simulink model "MainModel1"  (R2020a)
settings: Solver=FixedStepAuto  StartTime=0.0  StopTime=10  FixedStep=1e-3  RelTol=1e-3  EnableMultiTasking=on
undefined symbols (not defined in the file): A0, A3, D0, D1, D10, D11, D12, D13, D2, D3, D4, D5, D6, D7, D8, D9, PTA0, PTA1, PTA2, PTB11, PTB2, PTB23, PTB9, PTC16, PTC17, PTC2, PTC3, PTC4, PTD0, PTD1, PTD2, PTD3
libraries: frdmk64flib x17
settings Model: SimulationMode=external  ExtModeTrigDuration=5  Creator=prana  LastModifiedBy=prana
settings OptimizationCC: EnhancedBackFolding=on  PassReuseOutputArgsAs=Individual arguments  ZeroExternalMemoryAtStartup=off  ZeroInternalMemoryAtStartup=off  MaxStackSize=64  OptimizeBlockOrder=speed  DifferentSizesBufferReuse=on  OptimizationCustomize=off  EfficientTunableParamExpr=on
settings DebuggingCC: ParameterTunabilityLossMsg=error
settings HardwareCC: ProdBitPerPointer=32  ProdBitPerSizeT=32  ProdBitPerPtrDiffT=32  ProdLargestAtomicInteger=Long  ProdLargestAtomicFloat=Double  ProdWordSize=32  ProdHWDeviceType=ARM Compatible->ARM Cortex
settings SFSimCC: MATLABDynamicMemAlloc=off
settings RTWCC: SystemTargetFile=ert.tlc  HardwareBoard=NXP FRDM-K64F  TemplateMakefile=ert_default_tmf  Toolchain=GNU Tools for ARM Embedded Processors
settings CodeAppCC: ForceParamTrailComments=on  IgnoreCustomStorageClasses=off  OperatorAnnotations=on  SimulinkDataObjDesc=on  SFDataObjDesc=on  InsertBlockDesc=on

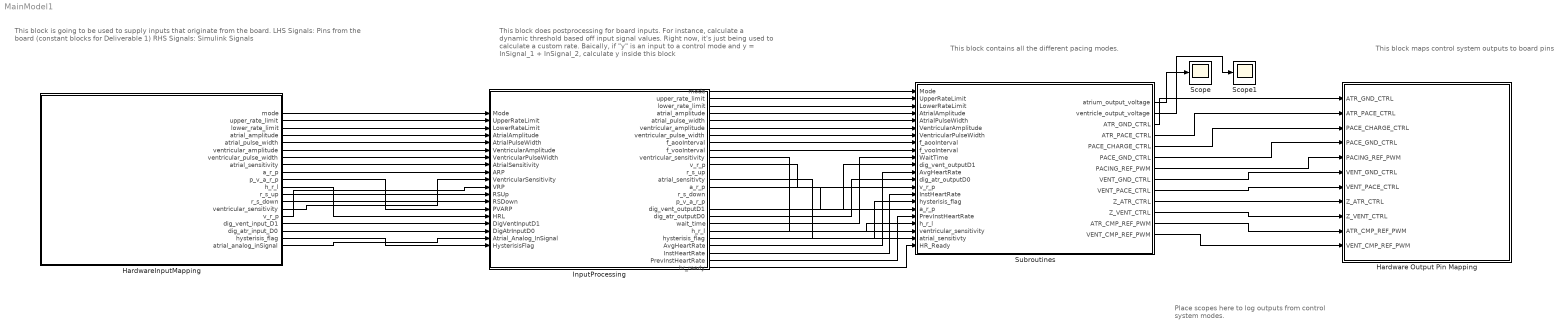
== system MainModel1 ==
  note: This block does postprocessing for board inputs.
      | For instance, calculate a dynamic threshold based off input signal values.
      | Right now, it's just being used to calculate a custom rate.
      | Baically, if "y" is an input to a control mode and y = InSignal_1 + InSignal_2,
      | calculate y inside this block
  note: This block is going to be used to supply inputs that originate from the board.
      | LHS Signals: Pins from the board (constant blocks for Deliverable 1)
      | RHS Signals: Simulink Signals
  note: This block contains all the different pacing modes.
  note: This block maps control system outputs to board pins
  note: Place scopes here to log outputs from control
      | system modes.
  Hardware Output Pin Mapping : Subsystem
  HardwareInputMapping : Subsystem
  InputProcessing : Subsystem
  Scope : Scope
  Scope1 : Scope
  Subroutines : Subsystem
  wires:
  InputProcessing/1(mode) -> Subroutines/1(Mode)
  InputProcessing/2(upper_rate_limit) -> Subroutines/2(UpperRateLimit)
  InputProcessing/3(lower_rate_limit) -> Subroutines/3(LowerRateLimit)
  InputProcessing/4(atrial_amplitude) -> Subroutines/4(AtrialAmplitude)
  InputProcessing/5(atrial_pulse_width) -> Subroutines/5(AtrialPulseWidth)
  InputProcessing/6(ventricular_amplitude) -> Subroutines/6(VentricularAmplitude)
  InputProcessing/7(ventricular_pulse_width) -> Subroutines/7(VentricularPulseWidth)
  InputProcessing/8(f_aooInterval) -> Subroutines/8(f_aooInterval)
  InputProcessing/9(f_vooInterval) -> Subroutines/9(f_vooInterval)
  Subroutines/1(atrium_output_voltage) -> Scope/1
  Subroutines/2(ventricle_output_voltage) -> Scope1/1
  HardwareInputMapping/1(mode) -> InputProcessing/1(Mode)
  HardwareInputMapping/2(upper_rate_limit) -> InputProcessing/2(UpperRateLimit)
  HardwareInputMapping/3(lower_rate_limit) -> InputProcessing/3(LowerRateLimit)
  HardwareInputMapping/4(atrial_amplitude) -> InputProcessing/4(AtrialAmplitude)
  HardwareInputMapping/5(atrial_pulse_width) -> InputProcessing/5(AtrialPulseWidth)
  HardwareInputMapping/6(ventricular_amplitude) -> InputProcessing/6(VentricularAmplitude)
  HardwareInputMapping/7(ventricular_pulse_width) -> InputProcessing/7(VentricularPulseWidth)
  HardwareInputMapping/8(atrial_sensitivity) -> InputProcessing/8(AtrialSensitivity)
  HardwareInputMapping/9(a_r_p) -> InputProcessing/9(ARP)
  HardwareInputMapping/14(ventricular_sensitivity) -> InputProcessing/10(VentricularSensitivity)
  HardwareInputMapping/15(v_r_p) -> InputProcessing/11(VRP)
  HardwareInputMapping/12(r_s_up) -> InputProcessing/12(RSUp)
  HardwareInputMapping/13(r_s_down) -> InputProcessing/13(RSDown)
  HardwareInputMapping/10(p_v_a_r_p) -> InputProcessing/14(PVARP)
  HardwareInputMapping/11(h_r_l) -> InputProcessing/15(HRL)
  HardwareInputMapping/16(dig_vent_input_D1) -> InputProcessing/16(DigVentInputD1)
  HardwareInputMapping/17(dig_atr_input_D0) -> InputProcessing/17(DigAtrInputD0)
  InputProcessing/19(wait_time) -> Subroutines/10(WaitTime)
  InputProcessing/17(dig_vent_outputD1) -> Subroutines/11(dig_vent_outputD1)
  InputProcessing/18(dig_atr_outputD0) -> Subroutines/13(dig_atr_outputD0)
  HardwareInputMapping/18(hysterisis_flag) -> InputProcessing/19(HysterisisFlag)
  HardwareInputMapping/19(atrial_analog_inSignal) -> InputProcessing/18(Atrial_Analog_InSignal)
  InputProcessing/22(AvgHeartRate) -> Subroutines/12(AvgHeartRate)
  InputProcessing/23(InstHeartRate) -> Subroutines/15(InstHeartRate)
  InputProcessing/21(hysterisis_flag) -> Subroutines/16(hysterisis_flag)
  InputProcessing/11(v_r_p) -> Subroutines/14(v_r_p)
  InputProcessing/14(a_r_p) -> Subroutines/17(a_r_p)
  InputProcessing/24(PrevInstHeartRate) -> Subroutines/18(PrevInstHeartRate)
  InputProcessing/20(h_r_l) -> Subroutines/19(h_r_l)
  Subroutines/3(ATR_GND_CTRL) -> Hardware Output Pin Mapping/1(ATR_GND_CTRL)
  Subroutines/4(ATR_PACE_CTRL) -> Hardware Output Pin Mapping/2(ATR_PACE_CTRL)
  Subroutines/5(PACE_CHARGE_CTRL) -> Hardware Output Pin Mapping/3(PACE_CHARGE_CTRL)
  Subroutines/6(PACE_GND_CTRL) -> Hardware Output Pin Mapping/4(PACE_GND_CTRL)
  Subroutines/7(PACING_REF_PWM) -> Hardware Output Pin Mapping/5(PACING_REF_PWM)
  Subroutines/8(VENT_GND_CTRL) -> Hardware Output Pin Mapping/6(VENT_GND_CTRL)
  Subroutines/9(VENT_PACE_CTRL) -> Hardware Output Pin Mapping/7(VENT_PACE_CTRL)
  Subroutines/10(Z_ATR_CTRL) -> Hardware Output Pin Mapping/8(Z_ATR_CTRL)
  Subroutines/11(Z_VENT_CTRL) -> Hardware Output Pin Mapping/9(Z_VENT_CTRL)
  InputProcessing/10(ventricular_sensitivity) -> Subroutines/20(ventricular_sensitivity)
  InputProcessing/13(atrial_sensitivty) -> Subroutines/21(atrial_sensitivty)
  Subroutines/12(ATR_CMP_REF_PWM) -> Hardware Output Pin Mapping/10(ATR_CMP_REF_PWM)
  Subroutines/13(VENT_CMP_REF_PWM) -> Hardware Output Pin Mapping/11(VENT_CMP_REF_PWM)
  InputProcessing/25(hr_ready) -> Subroutines/22(HR_Ready)

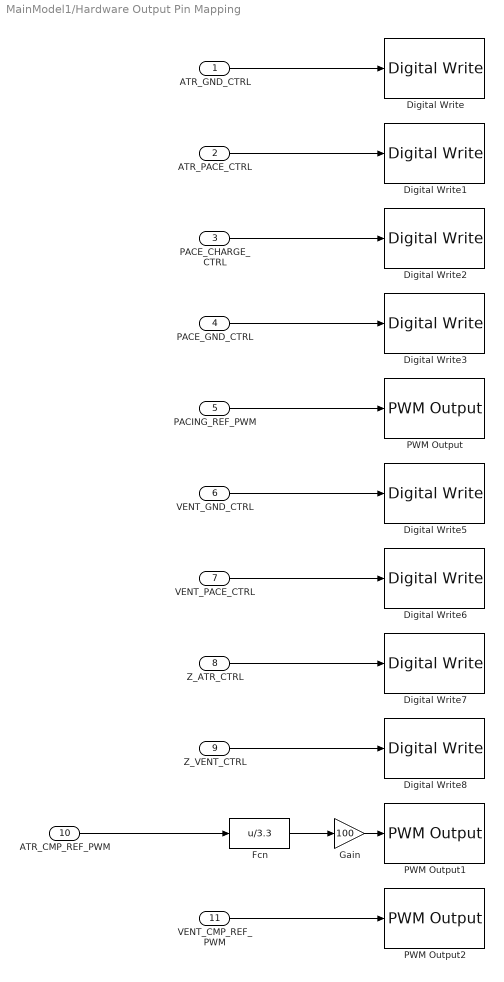
== system MainModel1/Hardware Output Pin Mapping ==
  ATR_GND_CTRL : Inport
  ATR_PACE_CTRL : Inport  Port=2
  PACE_CHARGE_CTRL : Inport  Port=3
  PACE_GND_CTRL : Inport  Port=4
  PACING_REF_PWM : Inport  Port=5
  VENT_GND_CTRL : Inport  Port=6
  VENT_PACE_CTRL : Inport  Port=7
  Z_ATR_CTRL : Inport  Port=8
  Z_VENT_CTRL : Inport  Port=9
  ATR_CMP_REF_PWM : Inport  Port=10
  VENT_CMP_REF_PWM : Inport  Port=11
  Digital Write : frdmk64flib/Digital Write  Whichpin=PTD2 (D11)
  Digital Write1 : frdmk64flib/Digital Write  Whichpin=PTA0 (D8)
  Digital Write2 : frdmk64flib/Digital Write  Whichpin=PTB9 (D2)
  Digital Write3 : frdmk64flib/Digital Write  Whichpin=PTD0 (D10)
  Digital Write5 : frdmk64flib/Digital Write  Whichpin=PTD3 (D12)
  Digital Write6 : frdmk64flib/Digital Write  Whichpin=PTC4 (D9)
  Digital Write7 : frdmk64flib/Digital Write  Whichpin=PTB23 (D4)
  Digital Write8 : frdmk64flib/Digital Write  Whichpin=PTC3 (D7)
  Fcn : Fcn  Expr=u/3.3
  Gain : Gain  Gain=100
  PWM Output : frdmk64flib/PWM Output  Whichpin=PTA2 (D5)  InitialFrequency=2000  InitialDutyCycle=100
  PWM Output1 : frdmk64flib/PWM Output  Whichpin=PTC2 (D6)  InitialFrequency=2000  InitialDutyCycle=20
  PWM Output2 : frdmk64flib/PWM Output  Whichpin=PTA1 (D3)  InitialFrequency=2000  InitialDutyCycle=20
  wires:
  ATR_GND_CTRL/1 -> Digital Write/1
  ATR_PACE_CTRL/1 -> Digital Write1/1
  PACE_CHARGE_CTRL/1 -> Digital Write2/1
  PACE_GND_CTRL/1 -> Digital Write3/1
  VENT_GND_CTRL/1 -> Digital Write5/1
  VENT_PACE_CTRL/1 -> Digital Write6/1
  Z_ATR_CTRL/1 -> Digital Write7/1
  Z_VENT_CTRL/1 -> Digital Write8/1
  PACING_REF_PWM/1 -> PWM Output/1
  VENT_CMP_REF_PWM/1 -> PWM Output2/1
  ATR_CMP_REF_PWM/1 -> Fcn/1
  Fcn/1 -> Gain/1
  Gain/1 -> PWM Output1/1

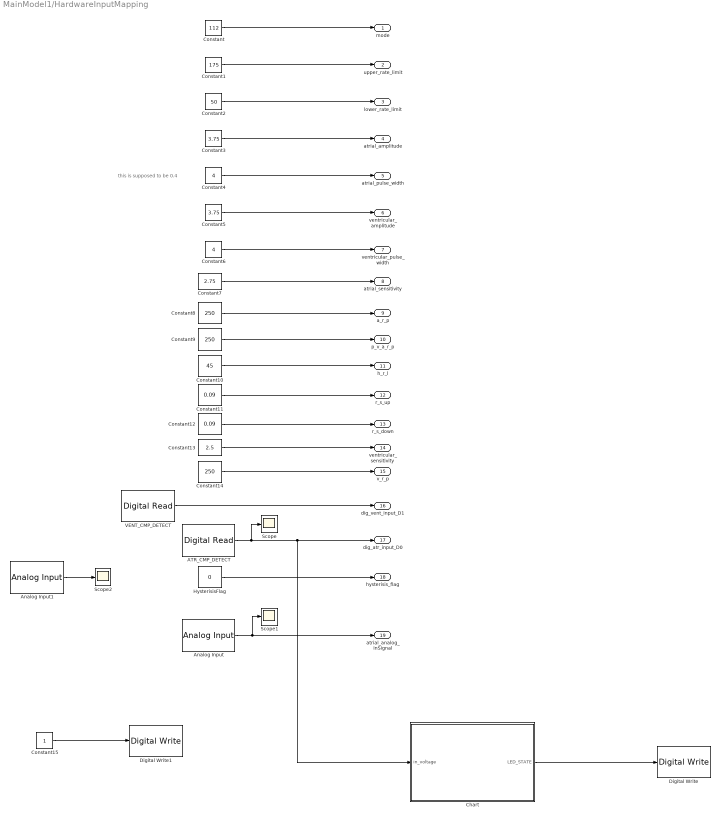
== system MainModel1/HardwareInputMapping ==
  note: this is supposed to be 0.4
  ATR_CMP_DETECT : frdmk64flib/Digital Read  Whichpin=PTC16 (D0)  SampleTime=0.001
  Analog Input : frdmk64flib/Analog Input  Whichpin=PTB2 (A0)  SampleTime=0.001
  Analog Input1 : frdmk64flib/Analog Input  Whichpin=PTB11 (A3)  SampleTime=0.001
  Chart : Stateflow chart  TreatAsAtomicUnit=on
  Constant : Constant  Value=112  OutDataTypeStr=uint32
  Constant1 : Constant  Value=175  OutDataTypeStr=uint32
  Constant10 : Constant  Value=45
  Constant11 : Constant  Value=0.09
  Constant12 : Constant  Value=0.09
  Constant13 : Constant  Value=2.5
  Constant14 : Constant  Value=250
  Constant15 : Constant  OutDataTypeStr=boolean
  Constant2 : Constant  Value=50  OutDataTypeStr=uint32
  Constant3 : Constant  Value=3.75  OutDataTypeStr=single
  Constant4 : Constant  Value=4  OutDataTypeStr=single
  Constant5 : Constant  Value=3.75  OutDataTypeStr=single
  Constant6 : Constant  Value=4  OutDataTypeStr=single
  Constant7 : Constant  Value=2.75
  Constant8 : Constant  Value=250
  Constant9 : Constant  Value=250
  Digital Write : frdmk64flib/Digital Write  Whichpin=RED_LED
  Digital Write1 : frdmk64flib/Digital Write  Whichpin=PTD1 (D13)
  HysterisisFlag : Constant  Value=0  OutDataTypeStr=boolean
  Scope : Scope
  Scope1 : Scope
  Scope2 : Scope
  VENT_CMP_DETECT : frdmk64flib/Digital Read  Whichpin=PTC17 (D1)  SampleTime=0.001
  mode : Outport  OutDataTypeStr=uint32
  upper_rate_limit : Outport  Port=2
  lower_rate_limit : Outport  Port=3
  atrial_amplitude : Outport  Port=4
  atrial_pulse_width : Outport  Port=5
  ventricular_amplitude : Outport  Port=6
  ventricular_pulse_width : Outport  Port=7
  atrial_sensitivity : Outport  Port=8
  a_r_p : Outport  Port=9
  p_v_a_r_p : Outport  Port=10
  h_r_l : Outport  Port=11
  r_s_up : Outport  Port=12
  r_s_down : Outport  Port=13
  ventricular_sensitivity : Outport  Port=14
  v_r_p : Outport  Port=15
  dig_vent_input_D1 : Outport  Port=16
  dig_atr_input_D0 : Outport  Port=17
  hysterisis_flag : Outport  Port=18
  atrial_analog_inSignal : Outport  Port=19
  wires:
  Constant/1 -> mode/1
  Constant1/1 -> upper_rate_limit/1
  Constant2/1 -> lower_rate_limit/1
  Constant3/1 -> atrial_amplitude/1
  Constant4/1 -> atrial_pulse_width/1
  Constant5/1 -> ventricular_amplitude/1
  Constant6/1 -> ventricular_pulse_width/1
  Constant8/1 -> a_r_p/1
  Constant9/1 -> p_v_a_r_p/1
  Constant10/1 -> h_r_l/1
  Constant11/1 -> r_s_up/1
  Constant12/1 -> r_s_down/1
  Constant13/1 -> ventricular_sensitivity/1
  Constant14/1 -> v_r_p/1
  ATR_CMP_DETECT/1 -> Scope/1, Chart/1(in_voltage), dig_atr_input_D0/1
  HysterisisFlag/1 -> hysterisis_flag/1
  Analog Input/1 -> Scope1/1, atrial_analog_inSignal/1
  VENT_CMP_DETECT/1 -> dig_vent_input_D1/1
  Chart/1(LED_STATE) -> Digital Write/1
  Constant15/1 -> Digital Write1/1
  Constant7/1 -> atrial_sensitivity/1
  Analog Input1/1 -> Scope2/1

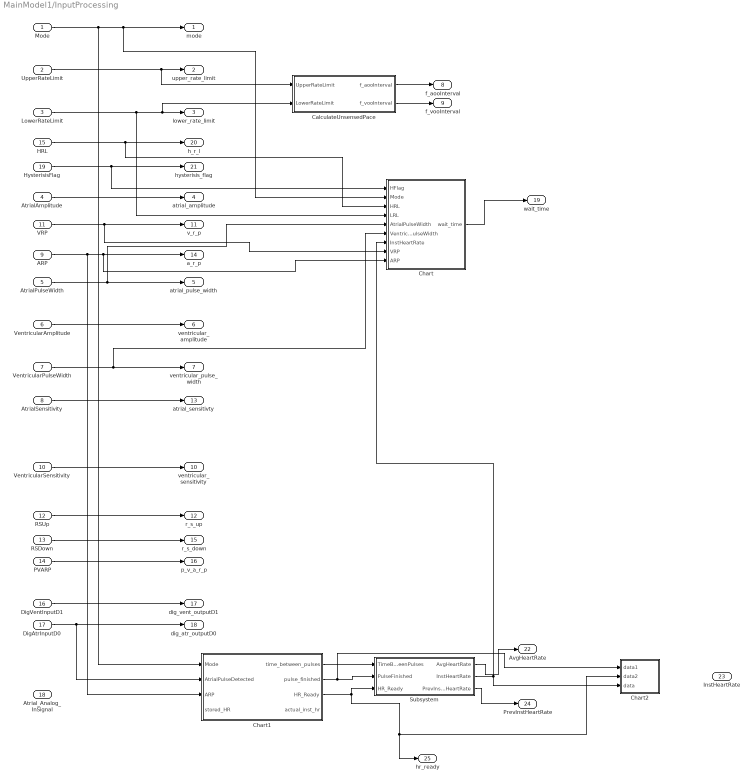
== system MainModel1/InputProcessing ==
  Mode : Inport
  UpperRateLimit : Inport  Port=2
  LowerRateLimit : Inport  Port=3
  AtrialAmplitude : Inport  Port=4
  AtrialPulseWidth : Inport  Port=5
  VentricularAmplitude : Inport  Port=6
  VentricularPulseWidth : Inport  Port=7
  AtrialSensitivity : Inport  Port=8
  ARP : Inport  Port=9
  VentricularSensitivity : Inport  Port=10
  VRP : Inport  Port=11
  RSUp : Inport  Port=12
  RSDown : Inport  Port=13
  PVARP : Inport  Port=14
  HRL : Inport  Port=15
  DigVentInputD1 : Inport  Port=16
  DigAtrInputD0 : Inport  Port=17
  Atrial_Analog_InSignal : Inport  Port=18
  HysterisisFlag : Inport  Port=19
  CalculateUnsensedPace : Subsystem
  Chart : Stateflow chart  TreatAsAtomicUnit=on
  Chart1 : Stateflow chart  TreatAsAtomicUnit=on
  Chart2 : Stateflow chart  TreatAsAtomicUnit=on
  Subsystem : Subsystem
  mode : Outport
  upper_rate_limit : Outport  Port=2
  lower_rate_limit : Outport  Port=3
  atrial_amplitude : Outport  Port=4
  atrial_pulse_width : Outport  Port=5
  ventricular_amplitude : Outport  Port=6
  ventricular_pulse_width : Outport  Port=7
  f_aooInterval : Outport  Port=8
  f_vooInterval : Outport  Port=9
  ventricular_sensitivity : Outport  Port=10
  v_r_p : Outport  Port=11
  r_s_up : Outport  Port=12
  atrial_sensitivty : Outport  Port=13
  a_r_p : Outport  Port=14
  r_s_down : Outport  Port=15
  p_v_a_r_p : Outport  Port=16
  dig_vent_outputD1 : Outport  Port=17
  dig_atr_outputD0 : Outport  Port=18
  wait_time : Outport  Port=19
  h_r_l : Outport  Port=20
  hysterisis_flag : Outport  Port=21
  AvgHeartRate : Outport  Port=22
  InstHeartRate : Outport  Port=23
  PrevInstHeartRate : Outport  Port=24
  hr_ready : Outport  Port=25
  wires:
  Mode/1 -> Chart1/1(Mode), Chart/2(Mode), mode/1
  UpperRateLimit/1 -> CalculateUnsensedPace/1(UpperRateLimit), upper_rate_limit/1
  LowerRateLimit/1 -> Chart/4(LRL), CalculateUnsensedPace/2(LowerRateLimit), lower_rate_limit/1
  AtrialAmplitude/1 -> atrial_amplitude/1
  AtrialPulseWidth/1 -> Chart/5(AtrialPulseWidth), atrial_pulse_width/1
  VentricularAmplitude/1 -> ventricular_amplitude/1
  VentricularPulseWidth/1 -> Chart/6(VentricularPulseWidth), ventricular_pulse_width/1
  CalculateUnsensedPace/1(f_aooInterval) -> f_aooInterval/1
  CalculateUnsensedPace/2(f_vooInterval) -> f_vooInterval/1
  VentricularSensitivity/1 -> ventricular_sensitivity/1
  VRP/1 -> Chart/8(VRP), v_r_p/1
  RSUp/1 -> r_s_up/1
  AtrialSensitivity/1 -> atrial_sensitivty/1
  ARP/1 -> Chart1/3(ARP), Chart/9(ARP), a_r_p/1
  RSDown/1 -> r_s_down/1
  PVARP/1 -> p_v_a_r_p/1
  HRL/1 -> Chart/3(HRL), h_r_l/1
  DigVentInputD1/1 -> dig_vent_outputD1/1
  DigAtrInputD0/1 -> Chart1/2(AtrialPulseDetected), dig_atr_outputD0/1
  HysterisisFlag/1 -> Chart/1(HFlag), hysterisis_flag/1
  Chart/1(wait_time) -> wait_time/1
  Chart1/1(time_between_pulses) -> Subsystem/1(TimeBetweenPulses)
  Chart1/2(pulse_finished) -> Chart2/1(data1), Subsystem/2(PulseFinished)
  Subsystem/1(AvgHeartRate) -> AvgHeartRate/1
  Subsystem/3(PrevInstHeartRate) -> PrevInstHeartRate/1
  Subsystem/2(InstHeartRate) -> Chart/7(InstHeartRate), Chart2/3(data)
  Chart1/3(HR_Ready) -> hr_ready/1, Chart2/2(data2), Subsystem/3(HR_Ready)

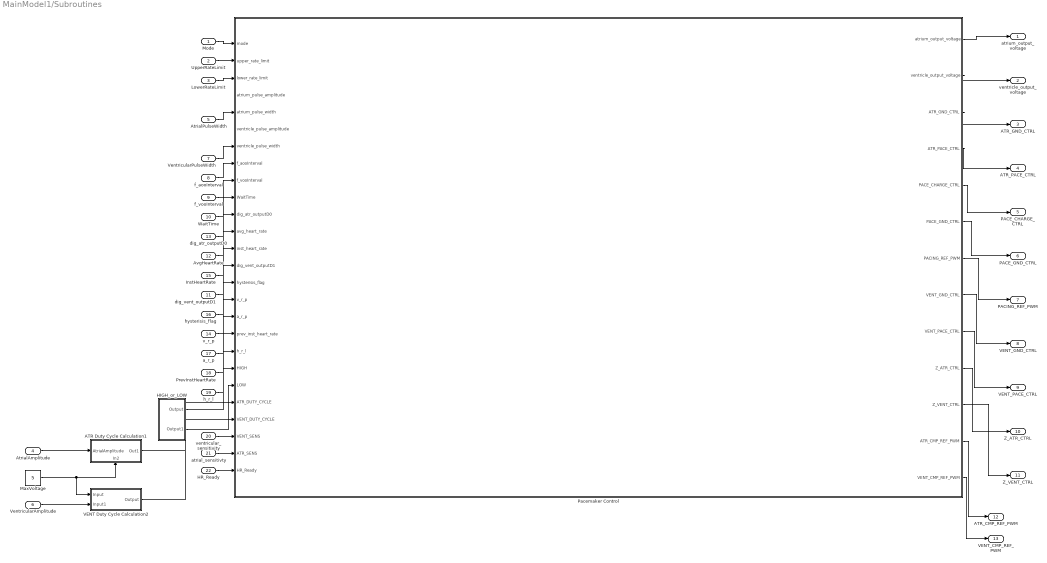
== system MainModel1/Subroutines ==
  Mode : Inport
  UpperRateLimit : Inport  Port=2
  LowerRateLimit : Inport  Port=3
  AtrialAmplitude : Inport  Port=4
  AtrialPulseWidth : Inport  Port=5
  VentricularAmplitude : Inport  Port=6
  VentricularPulseWidth : Inport  Port=7
  f_aooInterval : Inport  Port=8
  f_vooInterval : Inport  Port=9
  WaitTime : Inport  Port=10
  dig_vent_outputD1 : Inport  Port=11
  AvgHeartRate : Inport  Port=12
  dig_atr_outputD0 : Inport  Port=13
  v_r_p : Inport  Port=14
  InstHeartRate : Inport  Port=15
  hysterisis_flag : Inport  Port=16
  a_r_p : Inport  Port=17
  PrevInstHeartRate : Inport  Port=18
  h_r_l : Inport  Port=19
  ventricular_sensitivity : Inport  Port=20
  atrial_sensitivty : Inport  Port=21
  HR_Ready : Inport  Port=22
  ATR Duty Cycle Calculation1 : Subsystem
      settings: PortSchema="{\"entries\":[{\"content\":{\"sides\":[{\"content\":{\"connectorIds\":[\"In1\"]},\"type\":\"ConnectorPlacement.EquallySpacedRectSide\",\"uuid\":\"7d5ab2b8-d200-4a52-8dda-8470aabaf62e\"},{\"content\":{\"connectorIds\":[\"Out1\"],\"side\":\"RIGHT\"},\"type\":\"ConnectorPlacement.EquallySpacedRectSide\",\"uuid\":\"6eb8db6a-cd85-4876-a952-18d36bd2bab2\"},{\"content\":{\"connectorIds\":[],\"side\":\"TOP\"},\"type\":\"ConnectorPlacement.EquallySpacedRectSide\",\"uuid\":\"caadd8cd-4097-45ce-a5b0-5f06026e97cd\"},{\"content\":{\"connectorIds\":[\"In2\"],\"side\":\"BOTTOM\"},\"type\":\"ConnectorPlacement.EquallySpacedRectSide\",\"uuid\":\"bbb800c6-9a2c-47b7-a26a-3beb54eebb38\"}]},\"type\":\"ConnectorPlacement.EquallySpacedConnector\",\"uuid\":\"58b2cfcc-1743-4a3a-894e-e5458699235a\"}],\"packageUris\":[\"http://schema.mathworks.com/mf0/Connector/19700101\"],\"version\":\"1.0\"}"
  HIGH_or_LOW : Subsystem
      settings: PortSchema="{\"entries\":[{\"content\":{\"sides\":[{\"content\":{\"connectorIds\":[]},\"type\":\"ConnectorPlacement.EquallySpacedRectSide\",\"uuid\":\"49d8c1b3-c71d-4c5e-9f29-3a8fe0514842\"},{\"content\":{\"connectorIds\":[],\"side\":\"RIGHT\"},\"type\":\"ConnectorPlacement.EquallySpacedRectSide\",\"uuid\":\"0963f443-37bf-457e-bfcb-1d561403e5a9\"},{\"content\":{\"connectorIds\":[\"Out1\",\"Out2\"],\"side\":\"TOP\"},\"type\":\"ConnectorPlacement.EquallySpacedRectSide\",\"uuid\":\"32b78edd-16d0-4f55-b401-e4c12abc873e\"}]},\"type\":\"ConnectorPlacement.EquallySpacedConnector\",\"uuid\":\"974eb872-d95b-4224-a0e6-f13ce9826807\"}],\"packageUris\":[\"http://schema.mathworks.com/mf0/Connector/19700101\"],\"version\":\"1.0\"}"
  MaxVoltage : Constant  Value=5
  Pacemaker Control : Stateflow chart  TreatAsAtomicUnit=on
      settings: PortSchema="{\"entries\":[{\"content\":{\"sides\":[{\"content\":{\"connectorIds\":[\"In1\",\"In2\",\"In3\",\"In4\",\"In5\",\"In6\",\"In7\",\"In8\",\"In9\",\"In10\",\"In14\",\"In12\",\"In13\",\"In11\",\"In15\",\"In16\",\"In17\",\"In18\",\"In19\",\"In20\",\"In21\",\"In22\",\"In23\",\"In24\",\"In25\",\"In26\"]},\"type\":\"ConnectorPlacement.EquallySpacedRectSide\",\"uuid\":\"d7a0a1d4-1adb-4f49-9409-b65f2a410999\"},{\"content\":{\"connectorIds\":[\"Out1\",\"Out2\",\"Out3\",\"Out4\",\"Out5\",\"Out6\",\"Out7\",\"Out8\",\"Out9\",\"Out10\",\"Out11\",\"Out12\",\"Out13\"],\"side\":\"RIGHT\"},\"type\":\"ConnectorPlacement.EquallySpacedRectSide\",\"uuid\":\"f178eaad-70cd-4ec4-a78d-12af1cfbe493\"},{\"content\":{\"connectorIds\":[],\"side\":\"TOP\"},\"type\":\"ConnectorPlacement.EquallySpacedRectSide\",\"uuid\":\"df2c6513-3872-482b-abe5-5bf3da958119\"}]},\"type\":\"ConnectorPlacement.EquallySpacedConnector\",\"uuid\":\"0d6dffcb-0af9-47c5-9cde-377e88cba9d4\"}],\"packageUris\":[\"http://schema.mathworks.com/mf0/Connector/19700101\"],\"version\":\"1.0\"}"
  VENT Duty Cycle Calculation2 : Subsystem
  atrium_output_voltage : Outport
  ventricle_output_voltage : Outport  Port=2
  ATR_GND_CTRL : Outport  Port=3
  ATR_PACE_CTRL : Outport  Port=4
  PACE_CHARGE_CTRL : Outport  Port=5
  PACE_GND_CTRL : Outport  Port=6
  PACING_REF_PWM : Outport  Port=7
  VENT_GND_CTRL : Outport  Port=8
  VENT_PACE_CTRL : Outport  Port=9
  Z_ATR_CTRL : Outport  Port=10
  Z_VENT_CTRL : Outport  Port=11
  ATR_CMP_REF_PWM : Outport  Port=12
  VENT_CMP_REF_PWM : Outport  Port=13
  wires:
  Mode/1 -> Pacemaker Control/1(mode)
  Pacemaker Control/1(atrium_output_voltage) -> atrium_output_voltage/1
  Pacemaker Control/2(ventricle_output_voltage) -> ventricle_output_voltage/1
  UpperRateLimit/1 -> Pacemaker Control/2(upper_rate_limit)
  LowerRateLimit/1 -> Pacemaker Control/3(lower_rate_limit)
  AtrialPulseWidth/1 -> Pacemaker Control/5(atrium_pulse_width)
  VentricularPulseWidth/1 -> Pacemaker Control/7(ventricle_pulse_width)
  f_aooInterval/1 -> Pacemaker Control/8(f_aooInterval)
  f_vooInterval/1 -> Pacemaker Control/9(f_vooInterval)
  WaitTime/1 -> Pacemaker Control/10(WaitTime)
  dig_vent_outputD1/1 -> Pacemaker Control/11(dig_vent_outputD1)
  dig_atr_outputD0/1 -> Pacemaker Control/14(dig_atr_outputD0)
  AvgHeartRate/1 -> Pacemaker Control/12(avg_heart_rate)
  InstHeartRate/1 -> Pacemaker Control/13(inst_heart_rate)
  hysterisis_flag/1 -> Pacemaker Control/15(hysterisis_flag)
  v_r_p/1 -> Pacemaker Control/16(v_r_p)
  a_r_p/1 -> Pacemaker Control/17(a_r_p)
  PrevInstHeartRate/1 -> Pacemaker Control/18(prev_inst_heart_rate)
  h_r_l/1 -> Pacemaker Control/19(h_r_l)
  HIGH_or_LOW/1(Output) -> Pacemaker Control/20(HIGH)
  HIGH_or_LOW/2(Output1) -> Pacemaker Control/21(LOW)
  MaxVoltage/1 -> ATR Duty Cycle Calculation1/2(In2), VENT Duty Cycle Calculation2/1(Input)
  VentricularAmplitude/1 -> VENT Duty Cycle Calculation2/2(Input1)
  VENT Duty Cycle Calculation2/1(Output) -> Pacemaker Control/23(VENT_DUTY_CYCLE)
  AtrialAmplitude/1 -> ATR Duty Cycle Calculation1/1(AtrialAmplitude)
  ATR Duty Cycle Calculation1/1(Out1) -> Pacemaker Control/22(ATR_DUTY_CYCLE)
  Pacemaker Control/11(Z_VENT_CTRL) -> Z_VENT_CTRL/1
  Pacemaker Control/10(Z_ATR_CTRL) -> Z_ATR_CTRL/1
  Pacemaker Control/9(VENT_PACE_CTRL) -> VENT_PACE_CTRL/1
  Pacemaker Control/8(VENT_GND_CTRL) -> VENT_GND_CTRL/1
  Pacemaker Control/7(PACING_REF_PWM) -> PACING_REF_PWM/1
  Pacemaker Control/6(PACE_GND_CTRL) -> PACE_GND_CTRL/1
  Pacemaker Control/3(ATR_GND_CTRL) -> ATR_GND_CTRL/1
  Pacemaker Control/4(ATR_PACE_CTRL) -> ATR_PACE_CTRL/1
  Pacemaker Control/5(PACE_CHARGE_CTRL) -> PACE_CHARGE_CTRL/1
  ventricular_sensitivity/1 -> Pacemaker Control/24(VENT_SENS)
  atrial_sensitivty/1 -> Pacemaker Control/25(ATR_SENS)
  Pacemaker Control/12(ATR_CMP_REF_PWM) -> ATR_CMP_REF_PWM/1
  Pacemaker Control/13(VENT_CMP_REF_PWM) -> VENT_CMP_REF_PWM/1
  HR_Ready/1 -> Pacemaker Control/26(HR_Ready)

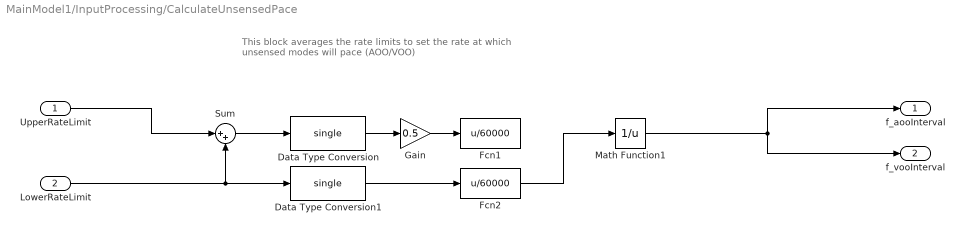
== system MainModel1/InputProcessing/CalculateUnsensedPace ==
  note: This block averages the rate limits to set the rate at which
      | unsensed modes will pace (AOO/VOO)
  UpperRateLimit : Inport
  LowerRateLimit : Inport  Port=2
  Data Type Conversion : DataTypeConversion  OutDataTypeStr=single
  Data Type Conversion1 : DataTypeConversion  OutDataTypeStr=single
  Fcn1 : Fcn  Expr=u/60000
  Fcn2 : Fcn  Expr=u/60000
  Gain : Gain  Gain=0.5
  Math Function1 : Math  Operator=reciprocal  SaturateOnIntegerOverflow=on
  Sum : Sum  Inputs=|++
  f_aooInterval : Outport
  f_vooInterval : Outport  Port=2
  wires:
  UpperRateLimit/1 -> Sum/1
  Math Function1/1 -> f_vooInterval/1, f_aooInterval/1
  Data Type Conversion1/1 -> Fcn2/1
  Gain/1 -> Fcn1/1
  Data Type Conversion/1 -> Gain/1
  Sum/1 -> Data Type Conversion/1
  Fcn2/1 -> Math Function1/1
  LowerRateLimit/1 -> Data Type Conversion1/1, Sum/2

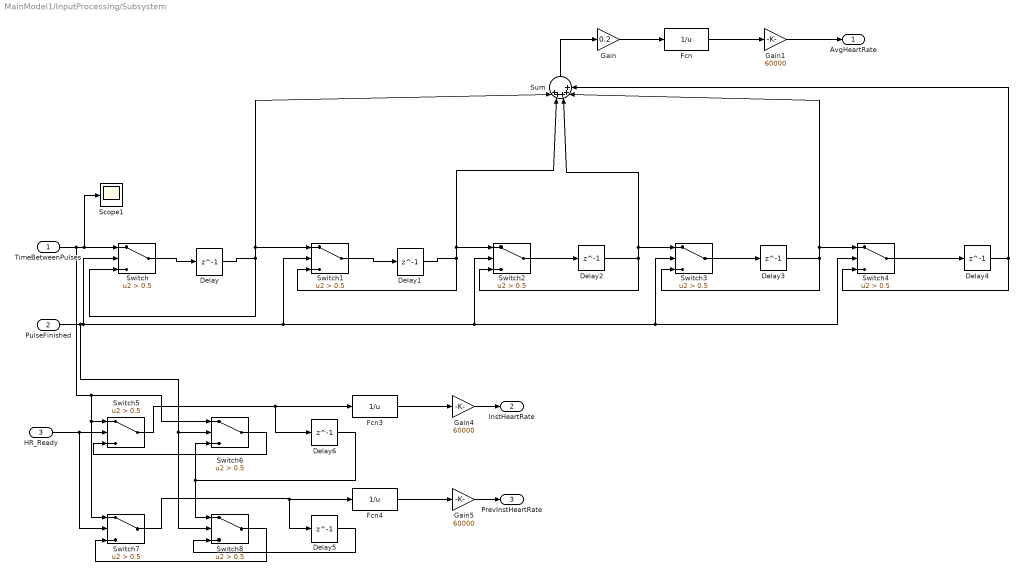
== system MainModel1/InputProcessing/Subsystem ==
  TimeBetweenPulses : Inport
  PulseFinished : Inport  Port=2
  HR_Ready : Inport  Port=3
  Delay{,1..4} (5 alike) : Delay  DelayLength=1
  Delay5 : Delay  DelayLength=1  SampleTime=0.001
  Delay6 : Delay  DelayLength=1  SampleTime=0.001
  Fcn : Fcn  Expr=1/u
  Fcn3 : Fcn  Expr=1/u
  Fcn4 : Fcn  Expr=1/u
  Gain : Gain  Gain=0.2
  Gain1 : Gain  Gain=60000
  Gain4 : Gain  Gain=60000
  Gain5 : Gain  Gain=60000
  Scope1 : Scope
  Sum : Sum  Inputs=|+++++
  Switch{,1..8} (9 alike) : Switch  Criteria=u2 > Threshold  Threshold=0.5
  AvgHeartRate : Outport
  InstHeartRate : Outport  Port=2
  PrevInstHeartRate : Outport  Port=3
  wires:
  Switch/1 -> Delay/1
  Switch1/1 -> Delay1/1
  Delay2/1 -> Sum/3, Switch3/1, Switch2/3
  Switch2/1 -> Delay2/1
  Delay3/1 -> Sum/4, Switch4/1, Switch3/3
  Switch3/1 -> Delay3/1
  Switch4/1 -> Delay4/1
  Delay4/1 -> Sum/5, Switch4/3
  Sum/1 -> Gain/1
  Gain/1 -> Fcn/1
  Fcn/1 -> Gain1/1
  Gain1/1 -> AvgHeartRate/1
  Delay/1 -> Sum/1, Switch1/1, Switch/3
  Delay1/1 -> Sum/2, Switch2/1, Switch1/3
  HR_Ready/1 -> Switch7/2, Switch5/2
  TimeBetweenPulses/1 -> Switch/1, Scope1/1, Switch5/1, Switch7/1, Switch6/1
  Switch5/1 -> Fcn3/1, Delay6/1
  PulseFinished/1 -> Switch4/2, Switch3/2, Switch2/2, Switch1/2, Switch/2, Switch8/2, Switch6/2
  Switch6/1 -> Switch5/3
  Delay6/1 -> Switch6/3, Switch8/1
  Switch8/1 -> Switch7/3
  Delay5/1 -> Switch8/3
  Switch7/1 -> Fcn4/1, Delay5/1
  Fcn3/1 -> Gain4/1
  Gain4/1 -> InstHeartRate/1
  Fcn4/1 -> Gain5/1
  Gain5/1 -> PrevInstHeartRate/1

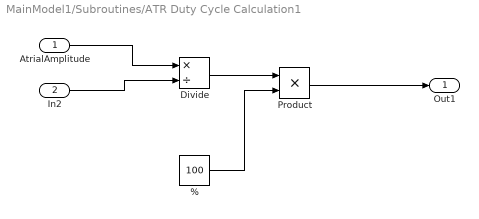
== system MainModel1/Subroutines/ATR Duty Cycle Calculation1 ==
  AtrialAmplitude : Inport
  In2 : Inport  Port=2
  % : Constant  Value=100
  Divide : Product  Inputs=*/
  Product : Product
  Out1 : Outport
  wires:
  Divide/1 -> Product/1
  %/1 -> Product/2
  AtrialAmplitude/1 -> Divide/1
  In2/1 -> Divide/2
  Product/1 -> Out1/1

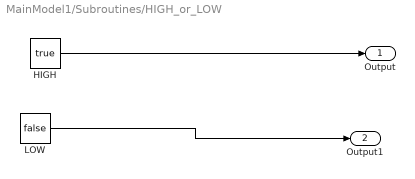
== system MainModel1/Subroutines/HIGH_or_LOW ==
  HIGH : Constant  Value=true
  LOW : Constant  Value=false
  Output : Outport
  Output1 : Outport  Port=2
  wires:
  LOW/1 -> Output1/1
  HIGH/1 -> Output/1

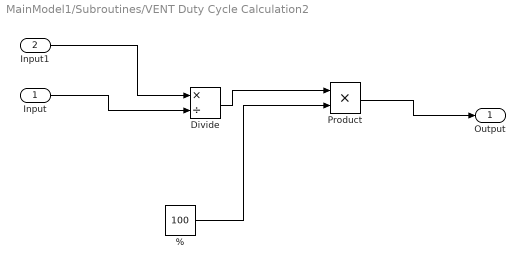
== system MainModel1/Subroutines/VENT Duty Cycle Calculation2 ==
  Input : Inport
  Input1 : Inport  Port=2
  % : Constant  Value=100
  Divide : Product  Inputs=*/
  Product : Product
  Output : Outport
  wires:
  Input/1 -> Divide/2
  Input1/1 -> Divide/1
  %/1 -> Product/2
  Divide/1 -> Product/1
  Product/1 -> Output/1

== stateflow chart MainModel1/InputProcessing/Chart ==
  state HysterisisSelection
    entry:
    time_minute = 60000; % ms/s
    smoothing_rate= InstHeartRate-5;
  state AAI
    entry:
    tot_wait_time = time_minute-((ARP+AtrialPulseWidth)*smoothing_rate);
    wait_time = tot_wait_time / smoothing_rate;
  state VVI
    entry:
    tot_wait_time = time_minute-((VRP+VentricularPulseWidth)*smoothing_rate);
    wait_time = tot_wait_time / smoothing_rate;
  (default) -> HysterisisSelection
  HysterisisSelection -> VVI [order 2] : [Mode==222]
  HysterisisSelection -> AAI [order 1] : [Mode==112]
  data: HFlag input; Mode input; HRL input; LRL input; AtrialPulseWidth input; VentricularPulseWidth input; InstHeartRate input; VRP input; ARP input; wait_time output; tot_wait_time local; time_minute local; smoothing_rate local

== stateflow chart MainModel1/InputProcessing/Chart2 ==
  state default
    entry
  (default) -> default
  data: data1 input; data2 input; data input

== stateflow chart MainModel1/Subroutines/Pacemaker Control ==
  state AAI
    state initializations
      entry:
      ATR_CMP_REF_PWM = ATR_SENS;
      %atrium_output_voltage  = 0;
      count=0;
    state Hysterisis_mode_ON
      entry:
      count = count +1;
    state Hysterisis_mode_OFF
      entry:
      count=count+1
    state Pulse
      entry:
      %atrium_output_voltage = atrium_pulse_amplitude;
      ATR_PACE_CTRL=LOW;
      VENT_PACE_CTRL=LOW;
      PACING_REF_PWM=ATR_DUTY_CYCLE;
      PACE_CHARGE_CTRL=HIGH;
      PACE_GND_CTRL=HIGH;
      Z_ATR_CTRL=LOW;
      Z_VENT_CTRL=LOW;
      ATR_GND_CTRL=HIGH;
      VENT_GND_CTRL=LOW;
    state ref1
      entry:
      %atrium_output_voltage = atrium_pulse_amplitude;
      PACE_CHARGE_CTRL=LOW;
      PACE_GND_CTRL=HIGH;
      ATR_PACE_CTRL=HIGH;
      ATR_GND_CTRL=LOW;
      Z_ATR_CTRL=LOW;
      Z_VENT_CTRL=LOW;
      VENT_GND_CTRL=LOW;
      VENT_PACE_CTRL=LOW;
      PACING_REF_PWM=ATR_DUTY_CYCLE;
    (default) -> AAI.initializations
    AAI.initializations -> AAI.Hysterisis_mode_ON [order 2] : [hysterisis_flag==1]
    AAI.initializations -> AAI.Hysterisis_mode_OFF [order 1] : [hysterisis_flag==0]
    AAI.Pulse -> AAI.initializations : [after(a_r_p,msec)]
    AAI.Hysterisis_mode_ON -> AAI.Hysterisis_mode_ON [order 2] : [(count<WaitTime)&&(~(dig_atr_outputD0 == LOW && inst_heart_rate<lower_rate_limit))]
    AAI.Hysterisis_mode_OFF -> AAI.Hysterisis_mode_OFF [order 1] : [(count<WaitTime)&&(~(dig_atr_outputD0 == LOW && inst_heart_rate<lower_rate_limit))]
    AAI.Hysterisis_mode_OFF -> AAI.ref1 [order 2] : [(dig_atr_outputD0 == LOW && inst_heart_rate<lower_rate_limit)||((count>WaitTime) && (dig_atr_outputD0 == LOW))]
    AAI.Hysterisis_mode_ON -> AAI.ref1 [order 1] : [(dig_atr_outputD0 == LOW && inst_heart_rate<h_r_l)||((count>WaitTime)&& (dig_atr_outputD0 == LOW))]
    AAI.ref1 -> AAI.Pulse : [after(atrium_pulse_width,msec)]
  state AOO
    state ChargeC22CapacitorandDischargeC21Capacitor
      entry:
      ATR_PACE_CTRL=LOW;
      VENT_PACE_CTRL=LOW;
      PACING_REF_PWM=ATR_DUTY_CYCLE;
      PACE_CHARGE_CTRL=HIGH;
      PACE_GND_CTRL=HIGH;
      Z_ATR_CTRL=LOW;
      Z_VENT_CTRL=LOW;
      ATR_GND_CTRL=HIGH;
      VENT_GND_CTRL=LOW;
      %atrium_output_voltage = atrium_pulse_amplitude;
      %exit:
      %atrium_output_voltage = 0;
    state PulseDISCHARGE
      entry:
      PACE_CHARGE_CTRL=LOW;
      PACE_GND_CTRL=HIGH;
      ATR_PACE_CTRL=HIGH;
      ATR_GND_CTRL=LOW;
      Z_ATR_CTRL=LOW;
      Z_VENT_CTRL=LOW;
      VENT_GND_CTRL=LOW;
      VENT_PACE_CTRL=LOW;
      PACING_REF_PWM=ATR_DUTY_CYCLE;
      %atrium_output_voltage = 0;
      %exit:
      %atrium_output_voltage = atrium_pulse_amplitude;
    (default) -> AOO.ChargeC22CapacitorandDischargeC21Capacitor
    PulseDISCHARGE -> AOO.ChargeC22CapacitorandDischargeC21Capacitor : [after(atrium_pulse_width,msec)]
    AOO.ChargeC22CapacitorandDischargeC21Capacitor -> PulseDISCHARGE : [after(f_aooInterval-atrium_pulse_width,msec)]
  state Initialize
    entry:
    AOO = 100;
    VOO = 200;
    AAI = 112;
    VVI = 222;
  state Standby
    entry:
    atrium_output_voltage = 0;
    ventricle_output_voltage = 0;
  state VOO
    state ChargeC22CapacitorandDischargeC21Capacitor
      entry:
      ATR_PACE_CTRL=LOW;
      VENT_PACE_CTRL=LOW;
      PACING_REF_PWM=VENT_DUTY_CYCLE;
      PACE_CHARGE_CTRL=HIGH;
      PACE_GND_CTRL=HIGH;
      Z_ATR_CTRL=LOW;
      Z_VENT_CTRL=LOW;
      ATR_GND_CTRL=LOW;
      VENT_GND_CTRL=HIGH;
      %atrium_output_voltage = atrium_pulse_amplitude;
      %exit:
      %atrium_output_voltage = 0;
    state StopPulseDISCHARGE
      entry:
      PACE_CHARGE_CTRL=LOW;
      PACE_GND_CTRL=HIGH;
      ATR_PACE_CTRL=LOW;
      ATR_GND_CTRL=LOW;
      Z_ATR_CTRL=LOW;
      Z_VENT_CTRL=LOW;
      VENT_GND_CTRL=LOW;
      VENT_PACE_CTRL=HIGH;
      PACING_REF_PWM=VENT_DUTY_CYCLE;
      %ventricle_output_voltage = 0;
      %exit:
      %ventricle_output_voltage = ventricle_pulse_amplitude;
    (default) -> VOO.ChargeC22CapacitorandDischargeC21Capacitor
    StopPulseDISCHARGE -> VOO.ChargeC22CapacitorandDischargeC21Capacitor : [after(ventricle_pulse_width,msec)]
    VOO.ChargeC22CapacitorandDischargeC21Capacitor -> StopPulseDISCHARGE : [after(f_vooInterval-ventricle_pulse_width,msec)]
  state VVI
    state initializations
      entry:
      VENT_CMP_REF_PWM = VENT_SENS;
      %ventricle_output_voltage  = 0;
      count=0;
    state Hysterisis_mode_OFF
      entry:
      count=count+1
    state Pulse
      entry:
      %ventricle_output_voltage = ventricle_pulse_amplitude;
      ATR_PACE_CTRL=LOW;
      VENT_PACE_CTRL=LOW;
      PACING_REF_PWM=VENT_DUTY_CYCLE;
      PACE_CHARGE_CTRL=HIGH;
      PACE_GND_CTRL=HIGH;
      Z_ATR_CTRL=LOW;
      Z_VENT_CTRL=LOW;
      ATR_GND_CTRL=LOW;
      VENT_GND_CTRL=HIGH;
    state Hysterisis_mode_ON
      entry:
      count = count +1;
    state ref1
      entry:
      %ventricle_output_voltage = ventricle_pulse_amplitude;
      PACE_CHARGE_CTRL=LOW;
      PACE_GND_CTRL=HIGH;
      ATR_PACE_CTRL=LOW;
      ATR_GND_CTRL=LOW;
      Z_ATR_CTRL=LOW;
      Z_VENT_CTRL=LOW;
      VENT_GND_CTRL=LOW;
      VENT_PACE_CTRL=HIGH;
      PACING_REF_PWM=VENT_DUTY_CYCLE;
    (default) -> VVI.initializations
    VVI.initializations -> VVI.Hysterisis_mode_ON [order 2] : [hysterisis_flag==1]
    VVI.initializations -> VVI.Hysterisis_mode_OFF [order 1] : [hysterisis_flag==0]
    VVI.Pulse -> VVI.initializations : [after(v_r_p,msec)]
    VVI.Hysterisis_mode_OFF -> VVI.Hysterisis_mode_OFF [order 1] : [(count<WaitTime)&&(~(dig_vent_outputD1 == LOW && inst_heart_rate<lower_rate_limit))]
    VVI.Hysterisis_mode_ON -> VVI.Hysterisis_mode_ON [order 2] : [(count<WaitTime)&&(~(dig_vent_outputD1 == LOW && inst_heart_rate<lower_rate_limit))]
    VVI.Hysterisis_mode_OFF -> VVI.ref1 [order 2] : [(dig_vent_outputD1 == LOW && inst_heart_rate<lower_rate_limit)||((count>WaitTime) && (dig_vent_outputD1 == LOW))]
    VVI.Hysterisis_mode_ON -> VVI.ref1 [order 1] : [(dig_vent_outputD1 == LOW && inst_heart_rate<h_r_l)||((count>WaitTime)&& (dig_vent_outputD1 == LOW))]
    VVI.ref1 -> VVI.Pulse : [after(ventricle_pulse_width,msec)]
  AOO -> Standby : [mode ~= AOO]
  Standby -> AOO [order 1] : [mode == AOO]
  AAI -> Standby : [mode ~= AAI]
  Standby -> AAI [order 4] : [mode == AAI]
  (default) -> Initialize
  Initialize -> Standby : [HR_Ready == true]
  VOO -> Standby : [mode ~= VOO]
  Standby -> VOO [order 3] : [mode == VOO]
  VVI -> Standby : [mode ~= VVI]
  Standby -> VVI [order 2] : [mode == VVI]
  data: mode input uint32; upper_rate_limit input uint32; lower_rate_limit input uint32; atrium_pulse_amplitude input single; atrium_pulse_width input single; ventricle_pulse_amplitude input single; ventricle_pulse_width input single; f_aooInterval input single; f_vooInterval input single; atrium_output_voltage output single; ventricle_output_voltage output single; AAI local uint32; VVI local uint32; VOO local int32; AOO local uint32; WaitTime input; dig_vent_outputD1 input; avg_heart_rate input; inst_heart_rate input; dig_atr_outputD0 input; hysterisis_flag input; v_r_p input; a_r_p input; prev_inst_heart_rate input; h_r_l input; count local; ATR_GND_CTRL output; ATR_PACE_CTRL output; PACE_CHARGE_CTRL output; PACE_GND_CTRL output; PACING_REF_PWM output; VENT_GND_CTRL output; VENT_PACE_CTRL output; Z_ATR_CTRL output; Z_VENT_CTRL output; HIGH input; LOW input; ATR_DUTY_CYCLE input; VENT_DUTY_CYCLE input; ATR_CMP_REF_PWM output; VENT_CMP_REF_PWM output; VENT_SENS input; ATR_SENS input; HR_Ready input boolean

== stateflow chart MainModel1/InputProcessing/Chart1 ==
  state default
    entry:
  state UnsensedModes
    entry:
    HR_Ready = true
    exit:
    HR_Ready = false
  state AtrialRateDetection
    state default
      entry:
      pulse_finished = 0
      time_between_pulses = 0
    state setARPasDeltaT
      entry:
      time_between_pulses = ARP
    state awaitNewPulse
      entry:
      time_between_pulses = time_between_pulses+1
    state newPulseDetected
      entry:
      pulse_finished = 1
      HR_Ready = true
    state resetDeltaT
      entry:
      pulse_finished = 0
      time_between_pulses = ARP
      actual_inst_hr = stored_HR
    (default) -> AtrialRateDetection.default
    AtrialRateDetection.default -> setARPasDeltaT : [AtrialPulseDetected == 1]
    setARPasDeltaT -> (junction 59) : [after(ARP,msec)]
    awaitNewPulse -> awaitNewPulse [order 1] : [AtrialPulseDetected == 0]
    (junction 59) -> awaitNewPulse [order 1] : [AtrialPulseDetected ==0]
    (junction 59) -> newPulseDetected [order 2] : [AtrialPulseDetected == 1]
    resetDeltaT -> (junction 59) : [after(ARP-1,msec)]
    awaitNewPulse -> newPulseDetected [order 2] : [AtrialPulseDetected == 1]
    newPulseDetected -> resetDeltaT : [after(1,msec)]
  (default) -> default
  default -> UnsensedModes [order 2] : [Mode == 100 || Mode == 200]
  UnsensedModes -> default : [Mode ~= 100 && Mode ~= 200]
  default -> AtrialRateDetection [order 1] : [Mode == 112]
  AtrialRateDetection -> default : [Mode ~= 112]
  data: Mode input; time_between_pulses output; pulse_finished output; AtrialPulseDetected input; ARP input; HR_Ready output boolean; stored_HR input; actual_inst_hr output

== stateflow chart MainModel1/HardwareInputMapping/Chart ==
  state default
    entry:
    LED_STATE = false
  note: 0.5,0.4,0.1,0.09,0.089,0.083,0.07, 0.05, 0.04, 0.039, 0.03, 0.02 worked
  note: 0.85, 0.95, 0.98, 0.99
  state led_on
    entry:
    LED_STATE = true
  (default) -> default
  default -> led_on : [in_voltage ==1]
  led_on -> default : [in_voltage ~= 1]
  data: LED_STATE output boolean; in_voltage input
